simulink model "untitled"  (Simulink 7.4)
settings: Solver=ode45  StartTime=0.0  StopTime=10.0  RelTol=1e-3
libraries: simulink x1
settings Model: Creator=autologin  LastModifiedBy=autologin

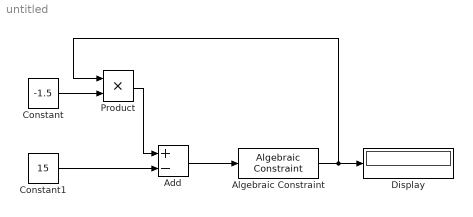
== system untitled ==
  Add : Sum  Inputs=+-  OutDataType=fixdt(1, 16)  OutScaling=2^-10
  Algebraic Constraint : simulink/Math Operations/Algebraic Constraint  SystemSampleTime=-1  z0=2
  Constant : Constant  Value=-1.5  OutDataType=fixdt(1, 16)  OutScaling=2^0
  Constant1 : Constant  Value=15  OutDataType=fixdt(1, 16)  OutScaling=2^0
  Display : Display
  Product : Product  OutDataType=fixdt(1, 16)  OutScaling=2^0  RndMeth=Zero
  wires:
  Constant1/1 -> Add/2
  Product/1 -> Add/1
  Algebraic Constraint/1 -> Display/1, Product/1
  Add/1 -> Algebraic Constraint/1
  Constant/1 -> Product/2
